simulink model "MRAS_IR2_Ld_Lq_simplified_inverter2"  (R2019b)
settings: Solver=ode23t  StartTime=0.0  StopTime=5  MaxStep=1e-6  RelTol=1e-3  EnableMultiTasking=on
libraries: powerlib x5, simulink x1
settings Model: Creator=Алексей  LastModifiedBy=Алексей
settings SolverCC: ZeroCrossControl=DisableAll  ZeroCrossAlgorithm=Adaptive
settings DataIOCC: SaveFormat=Array  SaveOutput=off  DSMLogging=off  SaveTime=off  ReturnWorkspaceOutputs=off
settings OptimizationCC: LifeSpan=inf
settings DebuggingCC: UnderspecifiedInitializationDetection=Classic  MergeDetectMultiDrivingBlocksExec=none  SolverPrmCheckMsg=warning  AllowSymbolicDim=off  SFUnexpectedBacktrackingDiag=warning  SFNoUnconditionalDefaultTransitionDiag=warning  SFExecutionAtInitializationDiag=none  ArithmeticOperatorsInVariantConditions=warning
settings HardwareCC: ProdBitPerPointer=32  ProdBitPerSizeT=32  ProdBitPerPtrDiffT=32  ProdLargestAtomicFloat=None  ProdIntDivRoundTo=Undefined  ProdEndianess=Unspecified  ProdWordSize=32  ProdHWDeviceType=32-bit Generic
settings ModelReferenceCC: PropagateSignalLabelsOutOfModel=off
settings SFSimCC: SimUseLocalCustomCode=off  CustomCodeUndefinedFunction=UseInterfaceOnly
settings RTWCC: RTWUseLocalCustomCode=off
settings CodeAppCC: StateflowObjectComments=on
settings GRTTargetCC: TargetLangStandard=C89/C90 (ANSI)  GeneratePreprocessorConditionals=Disable all
settings ConfigComp: CovMetricSettings=dw  CovHtmlReporting=on  CovSaveCumulativeToWorkspaceVar=on  CovSaveSingleToWorkspaceVar=on  CovExternalEMLEnable=off  CovSFcnEnable=off
settings SimscapeCC: SimscapeNormalizeSystem=off

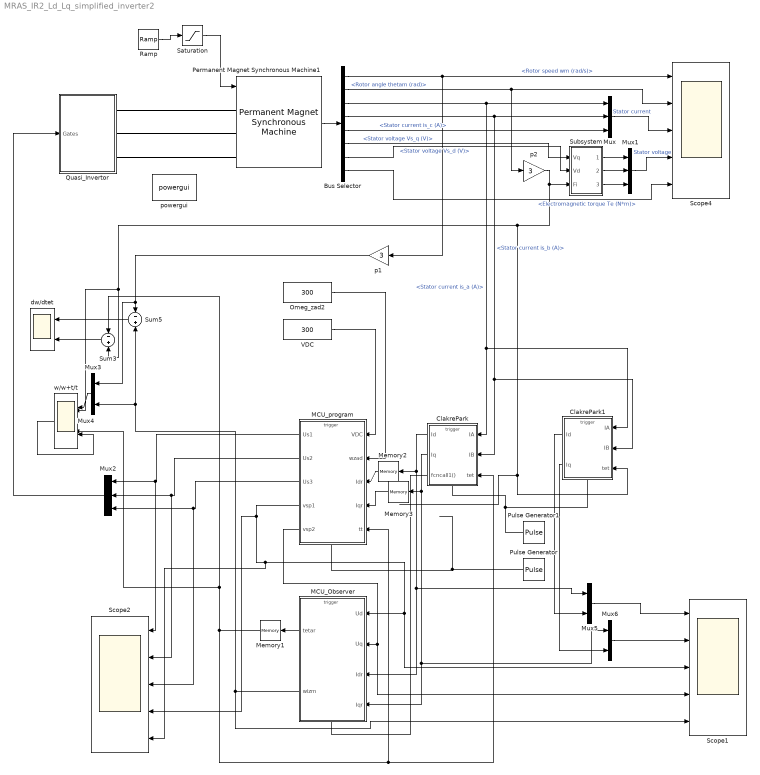
== system MRAS_IR2_Ld_Lq_simplified_inverter2 ==
  Bus Selector : BusSelector  OutputSignals=Rotor speed wm (rad/s),Rotor angle thetam (rad),Stator current is_a (A),Stator current is_b (A),Stator current is_c (A),Stator voltage Vs_q (V),Stator voltage Vs_d (V),Electromagnetic torque Te (N*m)
  ClakrePark : MATLAB Function  TreatAsAtomicUnit=on
  ClakrePark1 : MATLAB Function  TreatAsAtomicUnit=on
  MCU_Observer : MATLAB Function  TreatAsAtomicUnit=on
  MCU_program : MATLAB Function  TreatAsAtomicUnit=on
  Memory1 : Memory
  Memory2 : Memory
  Memory3 : Memory
  Mux : Mux  Inputs=3
  Mux1 : Mux  Inputs=3
  Mux2 : Mux  Inputs=3
  Mux{3..6} (4 alike) : Mux  Inputs=2
  Omeg_zad2 : Constant  Value=300
  Permanent Magnet Synchronous Machine1 : powerlib/Machines/Permanent Magnet Synchronous Machine  NbPhases=3  FluxDistribution=Sinusoidal  RotorType=Salient-pole  MechanicalLoad=Speed w  PresetModel=No  ShowDetailedParameters=on  MeasurementBus=off  Resistance=8  Inductance=8.5e-3  dqInductances=[21e-3,11e-3]  La=40e-3  MachineConstant=Flux linkage established by magnets (V.s)  Flux=0.157  VoltageCst=85.43  TorqueCst=0.7065  Flat=120  Mechanical=[2e-04 3e-03 3 0]  PolePairs=3  InitialConditions=[10,0, 0,0]  InitialConditions5ph=[0 0 0 0 0 0]  RefAngle=Aligned with phase A axis (original Park)  IterativeDiscreteModel=Trapezoidal non iterative  TsBlock=-1  TsPowergui=0
  Pulse Generator : DiscretePulseGenerator  PulseType=Time based  Period=100e-6  PulseWidth=10
  Pulse Generator1 : DiscretePulseGenerator  PulseType=Time based  Period=10e-6  PulseWidth=10
  Quasi_Invertor : Subsystem
  Ramp : simulink/Sources/Ramp  slope=300  start=0  InitialOutput=100
  Saturation : Saturate  UpperLimit=30  LowerLimit=0
  Scope1 : Scope  NumInputPorts=5
  Scope2 : Scope  NumInputPorts=5
  Scope4 : Scope  NumInputPorts=5
  Subsystem : Subsystem
  Sum3 : Sum  Inputs=-+
  Sum5 : Sum  Inputs=-+
  VDC : Constant  Value=300
  dw/dtet : Scope  NumInputPorts=2
  p1 : Gain  Gain=3
  p2 : Gain  Gain=3
  powergui : powerlib/powergui  Priority=1  SimulationMode=Continuous  SampleTime=50e-6  frequency=60  Iterations=50  frequencyindice=0  Pbase=100e6  ErrMax=1e-4  UnitsV=kV  UnitsW=MW  buscounter=0  FunctionMessages=off  echomessages=off  EnableUseOfTLC=off  CurrentSourceSwitches=on  DisableSnubberDevices=off  DisableRonSwitches=off  DisableVfSwitches=off  DisplayEquations=off  AutomaticDiscreteSolvers=off  SolverType=Tustin  Interpol=off  ExternalGateDelay=off  methode=off  Ts=0  x0status=blocks  SPID=off  SwTol=0  HookPort=off  NonlinearTolerance=1e-4  nMaxIteration=100  ContinueOnMaxIteration=off  RestoreLinks=warning  ResistiveCurrentMeasurement=off  Frange=[0:2:500]  Ylog=off  Xlog=on  ShowGrid=off  save=off  variable=ZData  structure=SD2  ZoomFFT=on  StartTime=0.7  cycles=10  DisplayStyle=4  fundamental=382  FreqAxis=off  MaxFrequency=50000  frequencyindicesteady=1  RmsSteady=1  display=off
      settings: SourceProductName=Simscape Electrical
  w/w+t/t : Scope  NumInputPorts=2
  wires:
  Bus Selector/3 -> Mux/1, ClakrePark1/1(IA), ClakrePark/1(IA)  "<Stator current is_a (A)>"
  Bus Selector/4 -> ClakrePark1/2(IB), ClakrePark/2(IB), Mux/2  "<Stator current is_b (A)>"
  Omeg_zad2/1 -> MCU_program/2(wzad)
  Permanent Magnet Synchronous Machine1/1 -> Bus Selector/1
  Bus Selector/5 -> Mux/3  "<Stator current is_c (A)>"
  Bus Selector/6 -> Subsystem/1(Vq)  "<Stator voltage Vs_q (V)>"
  Bus Selector/7 -> Subsystem/2(Vd)  "<Stator voltage Vs_d (V)>"
  Subsystem/2(Out2) -> Mux1/2
  Subsystem/3(Out3) -> Mux1/3
  Subsystem/1(Out1) -> Mux1/1
  Mux/1 -> Scope4/3  "Stator current"
  Mux1/1 -> Scope4/4  "Stator voltage"
  Bus Selector/8 -> Scope4/5  "<Electromagnetic torque Te (N*m)>"
  Sum3/1 -> dw/dtet/2
  Sum5/1 -> dw/dtet/1
  Saturation/1 -> Permanent Magnet Synchronous Machine1/1
  MCU_program/1(Us1) -> Scope2/1, Mux2/1
  MCU_program/2(Us2) -> Scope2/2, Mux2/2
  MCU_program/3(Us3) -> Scope2/3, Mux2/3
  Mux3/1 -> w/w+t/t/1
  Mux4/1 -> w/w+t/t/2
  Bus Selector/1 -> Scope4/1, p1/1  "<Rotor speed wm (rad/s)>"
  Bus Selector/2 -> p2/1, Scope4/2  "<Rotor angle thetam (rad)>"
  p2/1 -> ClakrePark1/3(tet), Mux4/1, Sum3/2, Subsystem/3(Fi)
  p1/1 -> Sum5/1, Mux3/1
  VDC/1 -> MCU_program/1(VDC)
  Mux2/1 -> Quasi_Invertor/1(Gates)
  MCU_program/5(vsp2) -> Scope1/4, MCU_Observer/2(Uq)
  MCU_program/4(vsp1) -> Scope2/5, Scope1/3, MCU_Observer/1(Ud), Scope2/4
  Pulse Generator/1 -> MCU_program/Trigger
  MCU_Observer/2(wizm) -> Scope1/5, Mux3/2, Sum5/2
  ClakrePark1/1(Id) -> Mux5/2
  ClakrePark1/2(Iq) -> Mux6/2
  Mux5/1 -> Scope1/1
  Mux6/1 -> Scope1/2
  ClakrePark/1(Id) -> Memory2/1, MCU_Observer/3(Idr), Mux5/1
  ClakrePark/2(Iq) -> MCU_Observer/4(Iqr), Mux6/1, Memory3/1
  Pulse Generator1/1 -> ClakrePark1/Trigger, ClakrePark/Trigger
  MCU_Observer/1(tetar) -> Memory1/1
  Ramp/1 -> Saturation/1
  ClakrePark/3(fcncall1()) -> MCU_Observer/Trigger
  ? -> ?
  Memory1/1 -> Mux4/2, Sum3/1, ClakrePark/3(tet), MCU_program/5(tt)
  Memory2/1 -> MCU_program/3(Idr)
  Memory3/1 -> MCU_program/4(Iqr)
  connections:
  Permanent Magnet Synchronous Machine1/LConn1 -- Quasi_Invertor/RConn1
  Quasi_Invertor/RConn3 -- Permanent Magnet Synchronous Machine1/LConn3
  Permanent Magnet Synchronous Machine1/LConn2 -- Quasi_Invertor/RConn2

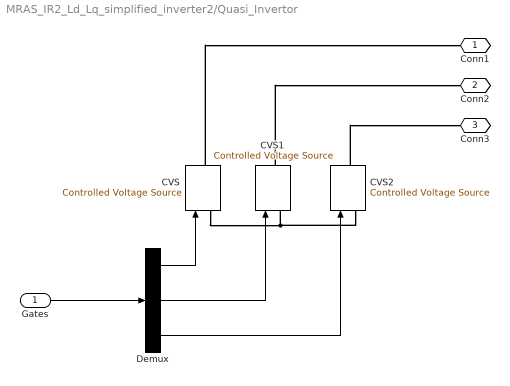
== system MRAS_IR2_Ld_Lq_simplified_inverter2/Quasi_Invertor ==
  Gates : Inport
  CVS : powerlib/Electrical Sources/Controlled Voltage Source  Initialize=on  Source_Type=AC  Amplitude=0  Phase=0  Frequency=0  Measurements=None
      settings: SourceProductName=Simscape Electrical
  CVS1 : powerlib/Electrical Sources/Controlled Voltage Source  Initialize=on  Source_Type=AC  Amplitude=0  Phase=0  Frequency=0  Measurements=None
      settings: SourceProductName=Simscape Electrical
  CVS2 : powerlib/Electrical Sources/Controlled Voltage Source  Initialize=on  Source_Type=AC  Amplitude=0  Phase=0  Frequency=0  Measurements=None
      settings: SourceProductName=Simscape Electrical
  Demux : Demux  Outputs=3
  Conn1 : PMIOPort  Side=Right
  Conn2 : PMIOPort  Port=2  Side=Right
  Conn3 : PMIOPort  Port=3  Side=Right
  wires:
  Demux/1 -> CVS/1
  Demux/2 -> CVS1/1
  Demux/3 -> CVS2/1
  Gates/1 -> Demux/1
  connections:
  CVS1/RConn1 -- Conn2/RConn1
  CVS2/RConn1 -- Conn3/RConn1
  CVS/RConn1 -- Conn1/RConn1
  CVS/LConn1 -- CVS2/LConn1 -- CVS1/LConn1

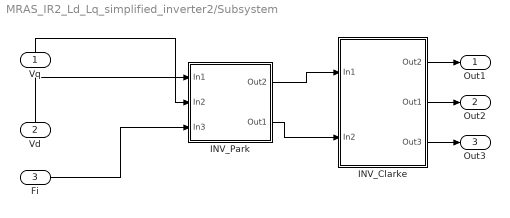
== system MRAS_IR2_Ld_Lq_simplified_inverter2/Subsystem ==
  Vq : Inport
  Vd : Inport  Port=2
  Fi : Inport  Port=3
  INV_Clarke : Subsystem
  INV_Park : Subsystem
  Out1 : Outport  VectorParamsAs1DForOutWhenUnconnected=off
  Out2 : Outport  Port=2  VectorParamsAs1DForOutWhenUnconnected=off
  Out3 : Outport  Port=3  VectorParamsAs1DForOutWhenUnconnected=off
  wires:
  INV_Clarke/2(Out1) -> Out2/1
  INV_Park/1(Out2) -> INV_Clarke/1(In1)
  INV_Clarke/1(Out2) -> Out1/1
  INV_Park/2(Out1) -> INV_Clarke/2(In2)
  INV_Clarke/3(Out3) -> Out3/1
  Fi/1 -> INV_Park/3(In3)
  Vd/1 -> INV_Park/1(In1)
  Vq/1 -> INV_Park/2(In2)

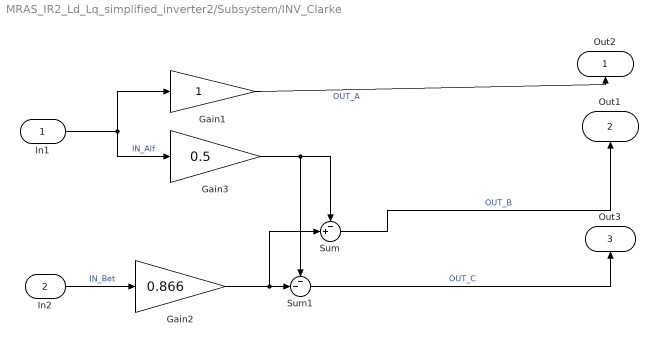
== system MRAS_IR2_Ld_Lq_simplified_inverter2/Subsystem/INV_Clarke ==
  In1 : Inport
  In2 : Inport  Port=2
  Gain1 : Gain
  Gain2 : Gain  Gain=0.866
  Gain3 : Gain  Gain=0.5
  Sum : Sum  Inputs=-+|
  Sum1 : Sum  Inputs=--|
  Out2 : Outport  VectorParamsAs1DForOutWhenUnconnected=off
  Out1 : Outport  Port=2  VectorParamsAs1DForOutWhenUnconnected=off
  Out3 : Outport  Port=3  VectorParamsAs1DForOutWhenUnconnected=off
  wires:
  Sum/1 -> Out1/1  "OUT_B"
  In2/1 -> Gain2/1  "IN_Bet"
  In1/1 -> Gain1/1, Gain3/1  "IN_Alf"
  Gain1/1 -> Out2/1  "OUT_A"
  Sum1/1 -> Out3/1  "OUT_C"
  Gain3/1 -> Sum1/1, Sum/1
  Gain2/1 -> Sum/2, Sum1/2

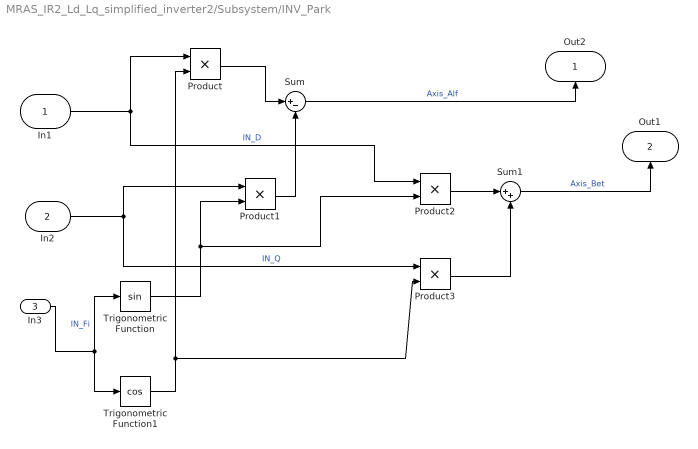
== system MRAS_IR2_Ld_Lq_simplified_inverter2/Subsystem/INV_Park ==
  In1 : Inport
  In2 : Inport  Port=2
  In3 : Inport  Port=3
  Product{,1..3} (4 alike) : Product
  Sum : Sum  Inputs=|+-
  Sum1 : Sum  Inputs=|++
  Trigonometric Function : Trigonometry
  Trigonometric Function1 : Trigonometry  Operator=cos
  Out2 : Outport  VectorParamsAs1DForOutWhenUnconnected=off
  Out1 : Outport  Port=2  VectorParamsAs1DForOutWhenUnconnected=off
  wires:
  Sum1/1 -> Out1/1  "Axis_Bet"
  In2/1 -> Product1/1, Product3/1  "IN_Q"
  In1/1 -> Product2/1, Product/1  "IN_D"
  Sum/1 -> Out2/1  "Axis_Alf"
  In3/1 -> Trigonometric Function1/1, Trigonometric Function/1  "IN_Fi"
  Trigonometric Function1/1 -> Product/2, Product3/2
  Trigonometric Function/1 -> Product2/2, Product1/2
  Product1/1 -> Sum/2
  Product/1 -> Sum/1
  Product2/1 -> Sum1/1
  Product3/1 -> Sum1/2

== matlab function MRAS_IR2_Ld_Lq_simplified_inverter2/MCU_Observer ==
  data: tetar output; Ud input; Uq input; Idr input; Iqr input; wizm output
  events: trigger input FUNCTION_CALL_EVENT
function [tetar,wizm] = fcn(Ud,Uq,Idr,Iqr)
%время 1/2 ШИМ периода
dt=10e-6;
%параметры машины
psi = 0.157;
R=8;
Ld=21e-3;
Lq=11e-3;


%Коэффициенты Пи-регулятора для МРАС
kint=350000;
kp=2.05;


persistent wrez;
persistent tetm;
persistent wint;
persistent Id; 
persistent Iq;

%заполнение начальных значений static переменным (persistent здесь)

if isempty(wrez)
    wrez=0;
end 
if isempty(tetm)
    tetm=0;
end 

if isempty(wint)
    wint=0;
end 
if isempty(Id)
    Id=0;
end   
if isempty(Iq)
    Iq=0;
end 

%------------------------------------------------------------------------------------------------------------
%Расчёт угла поворота через модель
%------------------------------------------------------------------------------------------------------------

                          
% производные нового шага для рассчётных значений токов Id и Iq
dId=-R/Ld*Id+wrez*Iq*Lq/Ld+Ud/Ld;
dIq=-wrez*Id*Ld/Lq-R/Lq*Iq-wrez*psi/Lq+Uq/Lq;
%рассчётные значения токов Id и Iq через производные 
Id=Id+dId*dt;
Iq=Iq+dIq*dt;
%реальные значения токов Id и Iq, полученные через  угол и оси альфа,бета 
%Idr=Ialfa*cos(tetm+wrez*dt)+Ibeta*sin(tetm+wrez*dt);
%Iqr=Ibeta*cos(tetm+wrez*dt)-Ialfa*sin(tetm+wrez*dt); 
%производная скорости через МРАС
dw=Idr*Iq-Iqr*Id-(Iqr-Iq)*psi/Ld;
%ПИ-регулятор МРАС
%интегральная составляющая
wint=wint+kint*dw*dt;
%пропорциональная составляющая
wp=dw*kp;
% результирующая П и И составяющая
wrez=wint+wp;
%Определение углового положения ротора по МРАС
tetm=tetm+wrez*dt;
tetar = tetm;
wizm = wrez;


return;

== matlab function MRAS_IR2_Ld_Lq_simplified_inverter2/ClakrePark ==
  data: IA input; IB input; Id output; tet input; Iq output
  events: trigger input RISING_EDGE_EVENT; fcncall1 output FUNCTION_CALL_EVENT
function [Id,Iq] = fcn(IA,IB,tet)

%Преобразование Кларка
Ialfa=IA;
Ibeta=(2*IB+IA)/1.7320508;

%реальные значения токов Id и Iq, полученные через  угол и оси альфа,бета 
Id=Ialfa*cos(tet)+Ibeta*sin(tet);
Iq=Ibeta*cos(tet)-Ialfa*sin(tet); 

fcncall1();
return;

== matlab function MRAS_IR2_Ld_Lq_simplified_inverter2/MCU_program ==
  data: VDC input; wzad input; Idr input; Iqr input; tt input; Us1 output; Us2 output; Us3 output; vsp1 output; vsp2 output
  events: trigger input RISING_EDGE_EVENT
function [Us1,Us2,Us3,vsp1,vsp2] = fcn(VDC,wzad,Idr,Iqr,tt)
dt = 100e-6;
R = 8;
Ld = 21e-3;
Lq = 11e-3;
persistent udint;
if (isempty(udint)) 
    udint = 20; 
end

persistent uqint;
if (isempty(uqint)) 
    uqint = 10; 
end

persistent Iqzad;
if (isempty(Iqzad)) 
    Iqzad = 0.1; 
end

kpq = 10;
kiq = kpq*R/Lq;

kpd = 10;
kid = kpd*R/Ld;

Idzad = 0;
Torque = 10;
%dTorque = Torque - wizm;
if (Iqzad<(Torque))
    Iqzad = Iqzad*1.05;
end

%Iqzad = Torque/1.5;%/3/psi;
dIq = Iqzad - Iqr;
dId = Idzad - Idr;

uqp = kpq* dIq;
uqint = uqint + kiq*dIq*dt;

udp = kpd* dId;
udint = udint + kid*dId*dt;

Uq = uqp + uqint;
Ud = udp + udint;

vrefa=sqrt(Uq^2+Ud^2);

if(vrefa>(2/3)*VDC)
  Ud=Ud*((2/3)*VDC/vrefa);
  Uq=Uq*((2/3)*VDC/vrefa);
end


Ua0=Ud*cos(tt)-Uq*sin(tt);
Ub0=Ud*sin(tt)+Uq*cos(tt);








%вывод на осциллографы



vsp1=Ud;
vsp2=Uq;



%алгоритм формирования фазных напряжений, КЛАРК


Us1=ceil(Ua0*100)/100;
Us2=sqrt(3)/2*Ub0-0.5*Ua0;
Us2=ceil(Us2*100)/100;
Us3=-0.5*Ua0-sqrt(3)/2*Ub0;
Us3=ceil(Us3*100)/100;




return;

== matlab function MRAS_IR2_Ld_Lq_simplified_inverter2/ClakrePark1 ==
  data: IA input; IB input; Id output; tet input; Iq output
  events: trigger input RISING_EDGE_EVENT
function [Id,Iq] = fcn(IA,IB,tet)

%Преобразование Кларка
Ialfa=IA;
Ibeta=(2*IB+IA)/1.7320508;

%реальные значения токов Id и Iq, полученные через  угол и оси альфа,бета 
Id=Ialfa*cos(tet)+Ibeta*sin(tet);
Iq=Ibeta*cos(tet)-Ialfa*sin(tet); 


return;
